simulink model "PR8_2"  (R2014b)
settings: Solver=ode45  StartTime=0.0  StopTime=10.0  RelTol=1e-3
libraries: simulink_extras x1
settings Model: Creator=Najmol Anwar  LastModifiedBy=Najmol Anwar

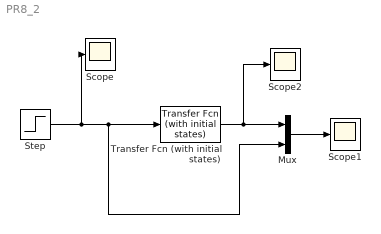
== system PR8_2 ==
  Mux : Mux  Inputs=2
  Scope : Scope
  Scope1 : Scope
  Scope2 : Scope
      settings: SaveName=ScopeData2
  Step : Step  SampleTime=0
  Transfer Fcn (with initial states) : simulink_extras/Additional Linear/Transfer Fcn (with initial states)  N=[1]  D="[1  5]"  X0=.5
  wires:
  Transfer Fcn (with initial states)/1 -> Scope2/1, Mux/1
  Mux/1 -> Scope1/1
  Step/1 -> Mux/2, Transfer Fcn (with initial states)/1, Scope/1
